simulink model "Cone_approach"  (R2024b)
settings: Solver=ode4  StartTime=0.0  StopTime=6000  FixedStep=0.01  RelTol=1e-3
values from neighbouring files (symbols this model uses):
  A = ly*lz    (= 0.25)    [Main.m]
  CD = 2.2    [Main.m]
  deltaVx_CA = 0.15    [Main.m]
  dp0_CA = dpf_RB    [Main.m]
  Dt = 0.01    [Main.m]
  Dt_con = 0.02    [Main.m]
  Dt_guid = 1    [Main.m]
  dx_max = 0.1    [Main.m]
  Ka = 1    [Main.m]
  kf = 4    [Main.m]
  landa_CA = 1.001    [Main.m]
  landa_CA_APF = 0.01    [Main.m]
  m_c0 = 50    [Main.m]
  omega_target = (mu/r_target^3)^0.5    (= 0.00113136572666)    [Main.m]
  p0_CA = pf_RB    [Main.m]
  pf_id = [-4 0 0]    [Main.m]
  rho = 1*10^(-12)    (= 1e-12)    [Main.m]
  S_CA = 0.35    [Main.m]
  S_CA_APF = 0.01    [Main.m]
  T1_CA = 10    [Main.m]
  T2_CA = T1_CA + deltax_CA/deltaVx_CA    [Main.m]
  tau = -ton/(log(1-(Uon-Uoff)/(Tmax*kf)))    [Main.m]
  Total_max_thrust = n*Tmax    (= 2)    [Main.m]
  Uoff = 0.7    [Main.m]
  Uon = 1    [Main.m]
  Vx = omega_target*r_target    (= 7668.56094333)    [Main.m]
undefined symbols (not defined in the file or in its folder): Fext
settings Model: Creator=corte  LastModifiedBy=aless

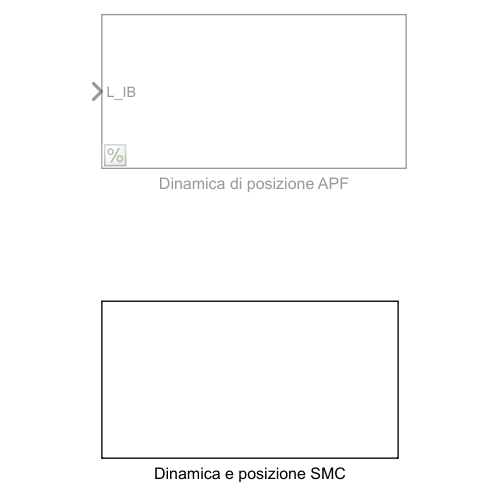
[thumbnail: Simulink's stored preview of the top-level diagram]
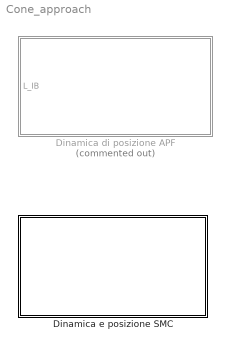
== system Cone_approach ==
  Dinamica di posizione APF : Subsystem  Commented=on
  Dinamica e posizione SMC : Subsystem

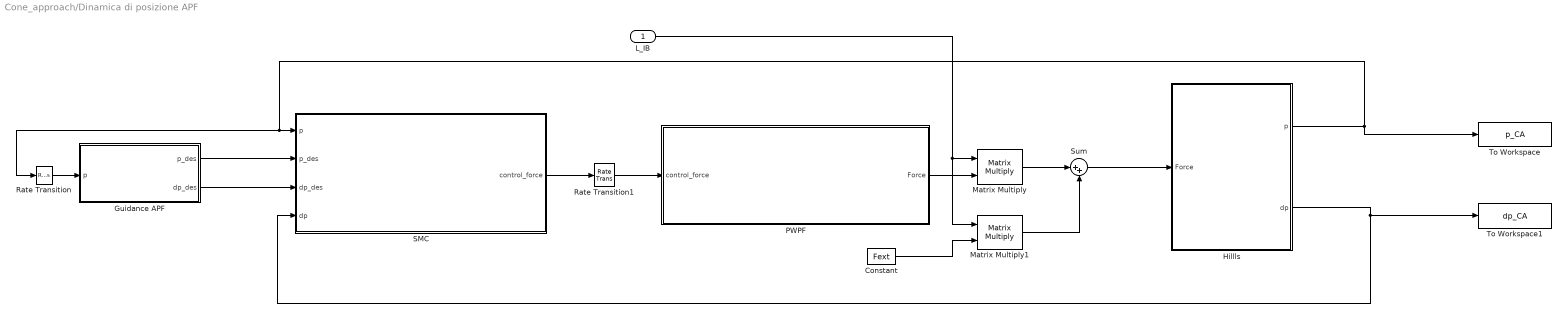
== system Cone_approach/Dinamica di posizione APF ==
  L_IB : Inport
  Constant : Constant  Value=Fext
  Guidance APF : Subsystem
  Hillls : Subsystem
  Matrix Multiply : Product  Multiplication=Matrix(*)
  Matrix Multiply1 : Product  Multiplication=Matrix(*)
  PWPF : Subsystem
  Rate Transition : RateTransition  InitialCondition=Dt  OutPortSampleTime=Dt_guid
  Rate Transition1 : RateTransition  InitialCondition=Dt_con  OutPortSampleTime=Dt
  SMC : Subsystem
  Sum : Sum  Inputs=|++
  To Workspace : ToWorkspace  VariableName=p_CA  SaveFormat=Timeseries  SampleTime=-1
  To Workspace1 : ToWorkspace  VariableName=dp_CA  SaveFormat=Timeseries  SampleTime=-1
  wires:
  Guidance APF/2(dp_des) -> SMC/3(dp_des)
  Hillls/1(p) -> To Workspace/1, Rate Transition/1, SMC/1(p)
  Guidance APF/1(p_des) -> SMC/2(p_des)
  Hillls/2(dp) -> SMC/4(dp), To Workspace1/1
  SMC/1(control_force) -> Rate Transition1/1
  Rate Transition/1 -> Guidance APF/1(p)
  Rate Transition1/1 -> PWPF/1(control_force)
  PWPF/1(Force) -> Matrix Multiply/2
  Matrix Multiply/1 -> Sum/1
  Sum/1 -> Hillls/1(Force)
  L_IB/1 -> Matrix Multiply1/1, Matrix Multiply/1
  Constant/1 -> Matrix Multiply1/2
  Matrix Multiply1/1 -> Sum/2

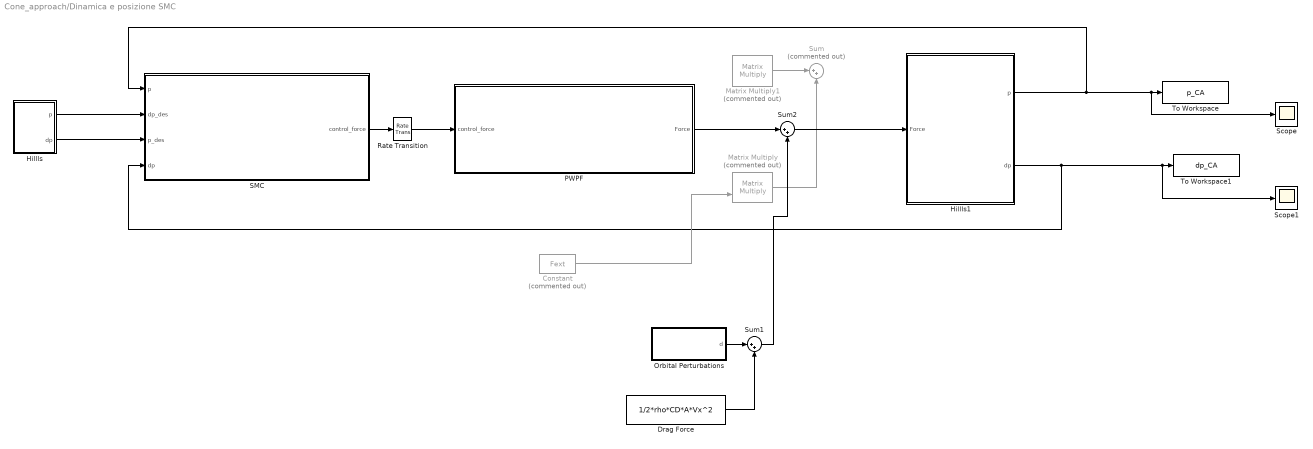
== system Cone_approach/Dinamica e posizione SMC ==
  Constant : Constant  Commented=on  Value=Fext
  Drag Force : Constant  Value=1/2*rho*CD*A*Vx^2
  Hillls : Subsystem
  Hillls1 : Subsystem
  Matrix Multiply : Product  Commented=on  Multiplication=Matrix(*)
  Matrix Multiply1 : Product  Commented=on  Multiplication=Matrix(*)
  Orbital Perturbations : Subsystem
  PWPF : Subsystem
  Rate Transition : RateTransition  InitialCondition=Dt_con  OutPortSampleTime=Dt_guid
  SMC : Subsystem
  Scope : Scope
  Scope1 : Scope
  Sum : Sum  Commented=on  Inputs=|++
  Sum1 : Sum  Inputs=|++
  Sum2 : Sum  Inputs=|++
  To Workspace : ToWorkspace  VariableName=p_CA  SaveFormat=Timeseries  SampleTime=-1
  To Workspace1 : ToWorkspace  VariableName=dp_CA  SaveFormat=Timeseries  SampleTime=-1
  wires:
  Hillls1/1(p) -> Scope/1, To Workspace/1, SMC/1(p)
  Hillls1/2(dp) -> Scope1/1, To Workspace1/1, SMC/4(dp)
  Hillls/1(p) -> SMC/2(dp_des)
  SMC/1(control_force) -> Rate Transition/1
  Hillls/2(dp) -> SMC/3(p_des)
  Rate Transition/1 -> PWPF/1(control_force)
  Constant/1 -> Matrix Multiply/2
  ? -> Matrix Multiply/1, Matrix Multiply1/1  "Aggiungere output controllo"
  Matrix Multiply/1 -> Sum/2
  Matrix Multiply1/1 -> Sum/1
  Sum1/1 -> Sum2/2
  Drag Force/1 -> Sum1/2
  Orbital Perturbations/1(d) -> Sum1/1
  PWPF/1(Force) -> Sum2/1
  Sum2/1 -> Hillls1/1(Force)

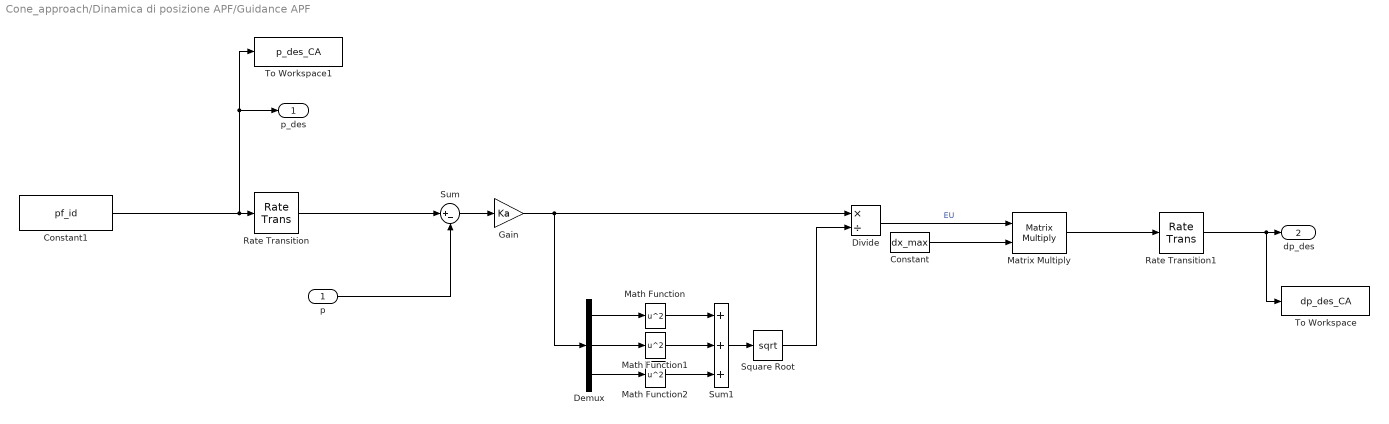
== system Cone_approach/Dinamica di posizione APF/Guidance APF ==
  p : Inport
  Constant : Constant  Value=dx_max
  Constant1 : Constant  Value=pf_id
  Demux : Demux  Outputs=3
  Divide : Product  Inputs=*/
  Gain : Gain  Gain=Ka
  Math Function : Math  Operator=square
  Math Function1 : Math  Operator=square
  Math Function2 : Math  Operator=square
  Matrix Multiply : Product  Multiplication=Matrix(*)
  Rate Transition : RateTransition  InitialCondition=Dt  OutPortSampleTime=Dt_guid
  Rate Transition1 : RateTransition  InitialCondition=Dt_guid  OutPortSampleTime=Dt
  Square Root : Sqrt
  Sum : Sum  Inputs=|+-
  Sum1 : Sum  Inputs=+++
  To Workspace : ToWorkspace  VariableName=dp_des_CA  SaveFormat=Timeseries  SampleTime=-1
  To Workspace1 : ToWorkspace  VariableName=p_des_CA  SaveFormat=Timeseries  SampleTime=-1
  p_des : Outport
  dp_des : Outport  Port=2
  wires:
  Sum/1 -> Gain/1
  p/1 -> Sum/2
  Rate Transition/1 -> Sum/1
  Constant1/1 -> To Workspace1/1, p_des/1, Rate Transition/1
  Gain/1 -> Demux/1, Divide/1
  Demux/1 -> Math Function/1
  Demux/2 -> Math Function1/1
  Demux/3 -> Math Function2/1
  Math Function/1 -> Sum1/1
  Math Function1/1 -> Sum1/2
  Math Function2/1 -> Sum1/3
  Sum1/1 -> Square Root/1
  Square Root/1 -> Divide/2
  Divide/1 -> Matrix Multiply/1  "EU"
  Constant/1 -> Matrix Multiply/2
  Matrix Multiply/1 -> Rate Transition1/1
  Rate Transition1/1 -> To Workspace/1, dp_des/1

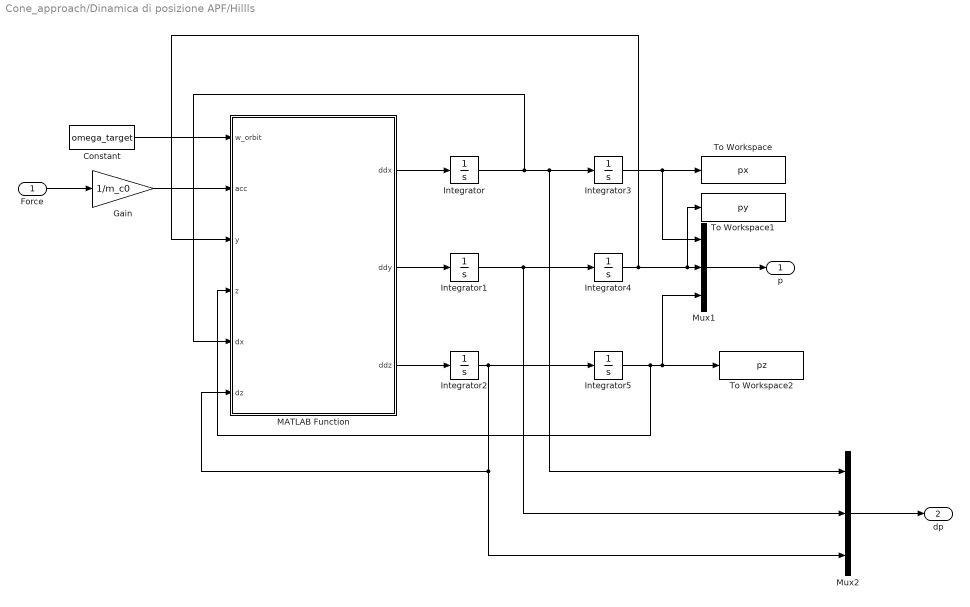
== system Cone_approach/Dinamica di posizione APF/Hillls ==
  Force : Inport
  Constant : Constant  Value=omega_target
  Gain : Gain  Gain=1/m_c0
  Integrator : Integrator  InitialCondition=dp0_CA(1)
  Integrator1 : Integrator  InitialCondition=dp0_CA(2)
  Integrator2 : Integrator  InitialCondition=dp0_CA(3)
  Integrator3 : Integrator  InitialCondition=p0_CA(1)
  Integrator4 : Integrator  InitialCondition=p0_CA(2)
  Integrator5 : Integrator  InitialCondition=p0_CA(3)
  MATLAB Function : MATLAB Function  TreatAsAtomicUnit=on
  Mux1 : Mux  Inputs=3
  Mux2 : Mux  Inputs=3
  To Workspace : ToWorkspace  VariableName=px  SaveFormat=Timeseries  SampleTime=-1
  To Workspace1 : ToWorkspace  VariableName=py  SaveFormat=Timeseries  SampleTime=-1
  To Workspace2 : ToWorkspace  VariableName=pz  SaveFormat=Timeseries  SampleTime=-1
  p : Outport
  dp : Outport  Port=2
  wires:
  Force/1 -> Gain/1
  Gain/1 -> MATLAB Function/2(acc)
  Constant/1 -> MATLAB Function/1(w_orbit)
  MATLAB Function/1(ddx) -> Integrator/1
  Integrator4/1 -> To Workspace1/1, Mux1/2, MATLAB Function/3(y)
  Integrator3/1 -> Mux1/1, To Workspace/1
  Integrator5/1 -> To Workspace2/1, Mux1/3, MATLAB Function/4(z)
  Integrator2/1 -> Integrator5/1, Mux2/3, MATLAB Function/6(dz)
  Integrator/1 -> Mux2/1, Integrator3/1, MATLAB Function/5(dx)
  MATLAB Function/2(ddy) -> Integrator1/1
  Integrator1/1 -> Mux2/2, Integrator4/1
  MATLAB Function/3(ddz) -> Integrator2/1
  Mux1/1 -> p/1
  Mux2/1 -> dp/1

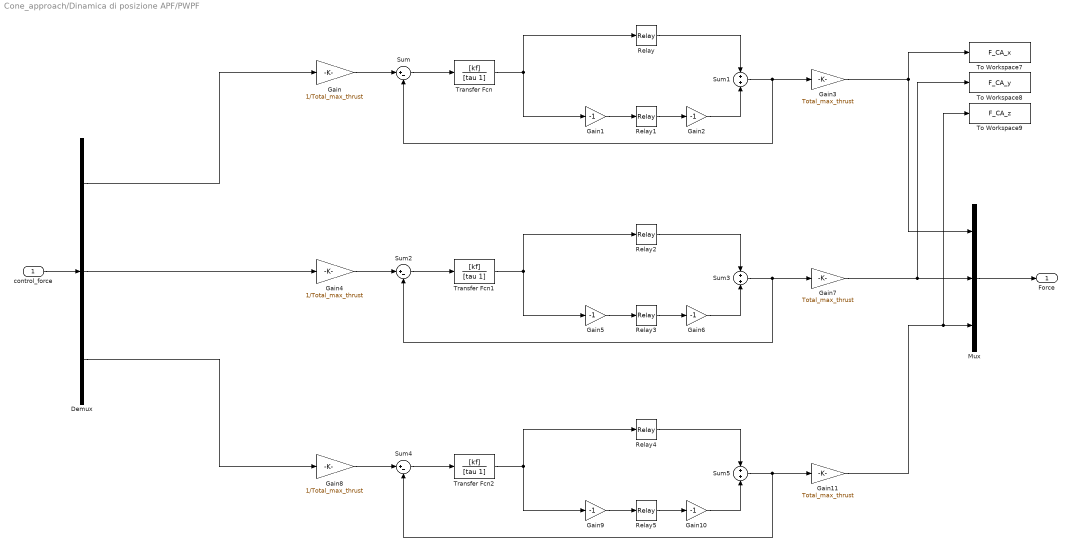
== system Cone_approach/Dinamica di posizione APF/PWPF ==
  control_force : Inport
  Demux : Demux  Outputs=3
  Gain : Gain  Gain=1/Total_max_thrust
  Gain{1..2,5..6,9..10} (6 alike) : Gain  Gain=-1
  Gain11 : Gain  Gain=Total_max_thrust
  Gain3 : Gain  Gain=Total_max_thrust
  Gain4 : Gain  Gain=1/Total_max_thrust
  Gain7 : Gain  Gain=Total_max_thrust
  Gain8 : Gain  Gain=1/Total_max_thrust
  Mux : Mux  Inputs=3
  Relay{,1..5} (6 alike) : Relay  OnSwitchValue=Uon  OffSwitchValue=Uoff
  Sum : Sum  Inputs=|+-
  Sum1 : Sum
  Sum2 : Sum  Inputs=|+-
  Sum3 : Sum
  Sum4 : Sum  Inputs=|+-
  Sum5 : Sum
  To Workspace7 : ToWorkspace  VariableName=F_CA_x  SaveFormat=Timeseries  SampleTime=-1
  To Workspace8 : ToWorkspace  VariableName=F_CA_y  SaveFormat=Timeseries  SampleTime=-1
  To Workspace9 : ToWorkspace  VariableName=F_CA_z  SaveFormat=Timeseries  SampleTime=-1
  Transfer Fcn : TransferFcn  Numerator=[kf]  Denominator=[tau 1]
  Transfer Fcn1 : TransferFcn  Numerator=[kf]  Denominator=[tau 1]
  Transfer Fcn2 : TransferFcn  Numerator=[kf]  Denominator=[tau 1]
  Force : Outport
  wires:
  Gain/1 -> Sum/1
  Gain1/1 -> Relay1/1
  Relay1/1 -> Gain2/1
  Relay/1 -> Sum1/1
  Gain2/1 -> Sum1/2
  Sum1/1 -> Sum/2, Gain3/1
  Sum/1 -> Transfer Fcn/1
  Transfer Fcn/1 -> Gain1/1, Relay/1
  control_force/1 -> Demux/1
  Demux/1 -> Gain/1
  Sum3/1 -> Sum2/2, Gain7/1
  Relay3/1 -> Gain6/1
  Gain5/1 -> Relay3/1
  Relay2/1 -> Sum3/1
  Gain4/1 -> Sum2/1
  Transfer Fcn1/1 -> Gain5/1, Relay2/1
  Demux/2 -> Gain4/1
  Sum2/1 -> Transfer Fcn1/1
  Gain6/1 -> Sum3/2
  Sum5/1 -> Sum4/2, Gain11/1
  Relay5/1 -> Gain10/1
  Gain9/1 -> Relay5/1
  Relay4/1 -> Sum5/1
  Gain8/1 -> Sum4/1
  Transfer Fcn2/1 -> Gain9/1, Relay4/1
  Demux/3 -> Gain8/1
  Sum4/1 -> Transfer Fcn2/1
  Gain10/1 -> Sum5/2
  Mux/1 -> Force/1
  Gain7/1 -> To Workspace8/1, Mux/2
  Gain3/1 -> To Workspace7/1, Mux/1
  Gain11/1 -> To Workspace9/1, Mux/3

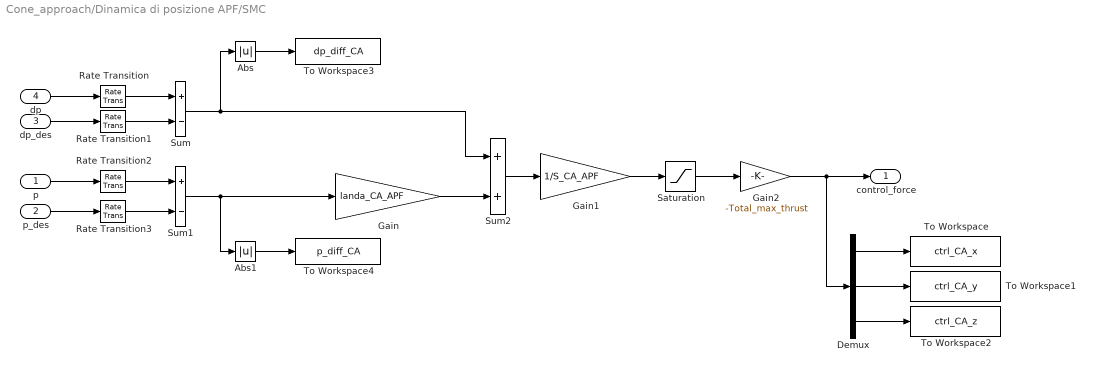
== system Cone_approach/Dinamica di posizione APF/SMC ==
  p : Inport
  p_des : Inport  Port=2
  dp_des : Inport  Port=3
  dp : Inport  Port=4
  Abs : Abs  SaturateOnIntegerOverflow=off
  Abs1 : Abs  SaturateOnIntegerOverflow=off
  Demux : Demux  Outputs=3
  Gain : Gain  Gain=landa_CA_APF
  Gain1 : Gain  Gain=1/S_CA_APF
  Gain2 : Gain  Gain=-Total_max_thrust
  Rate Transition{,1..3} (4 alike) : RateTransition  InitialCondition=Dt  OutPortSampleTime=Dt_con
  Saturation : Saturate  UpperLimit=1  LowerLimit=-1
  Sum : Sum  Inputs=+-
  Sum1 : Sum  Inputs=+-
  Sum2 : Sum
  To Workspace : ToWorkspace  VariableName=ctrl_CA_x  SaveFormat=Timeseries  SampleTime=-1
  To Workspace1 : ToWorkspace  VariableName=ctrl_CA_y  SaveFormat=Timeseries  SampleTime=-1
  To Workspace2 : ToWorkspace  VariableName=ctrl_CA_z  SaveFormat=Timeseries  SampleTime=-1
  To Workspace3 : ToWorkspace  VariableName=dp_diff_CA  SaveFormat=Timeseries  SampleTime=-1
  To Workspace4 : ToWorkspace  VariableName=p_diff_CA  SaveFormat=Timeseries  SampleTime=-1
  control_force : Outport
  wires:
  dp/1 -> Rate Transition/1
  dp_des/1 -> Rate Transition1/1
  p/1 -> Rate Transition2/1
  p_des/1 -> Rate Transition3/1
  Sum1/1 -> Abs1/1, Gain/1
  Gain/1 -> Sum2/2
  Sum/1 -> Abs/1, Sum2/1
  Sum2/1 -> Gain1/1
  Gain1/1 -> Saturation/1
  Saturation/1 -> Gain2/1
  Gain2/1 -> control_force/1, Demux/1
  Rate Transition/1 -> Sum/1
  Rate Transition1/1 -> Sum/2
  Rate Transition2/1 -> Sum1/1
  Rate Transition3/1 -> Sum1/2
  Demux/1 -> To Workspace/1
  Demux/2 -> To Workspace1/1
  Demux/3 -> To Workspace2/1
  Abs/1 -> To Workspace3/1
  Abs1/1 -> To Workspace4/1

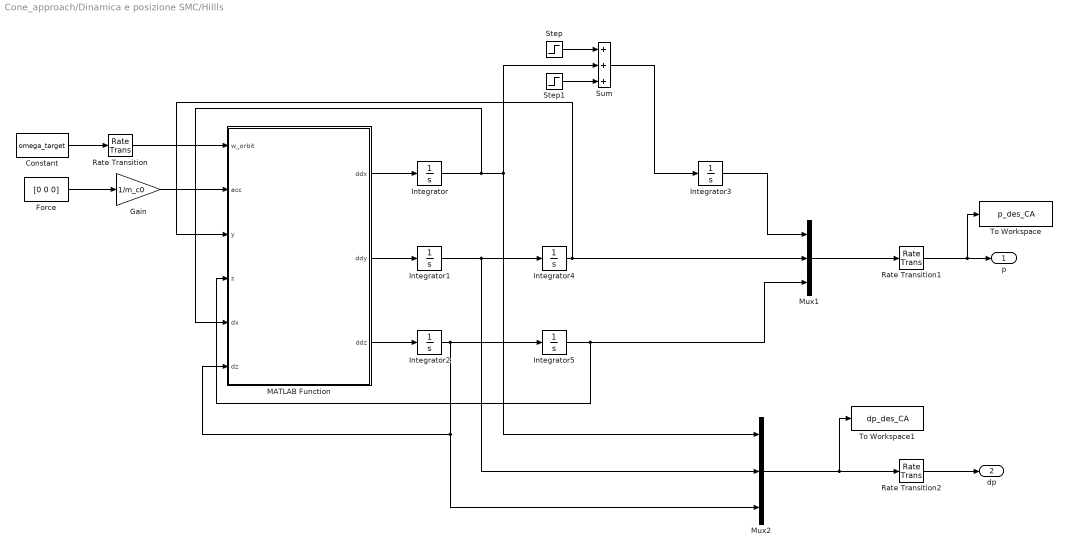
== system Cone_approach/Dinamica e posizione SMC/Hillls ==
  Constant : Constant  Value=omega_target
  Force : Constant  Value=[0 0 0]
  Gain : Gain  Gain=1/m_c0
  Integrator : Integrator  InitialCondition=dp0_CA(1)
  Integrator1 : Integrator  InitialCondition=dp0_CA(2)
  Integrator2 : Integrator  InitialCondition=dp0_CA(3)
  Integrator3 : Integrator  InitialCondition=p0_CA(1)
  Integrator4 : Integrator  InitialCondition=p0_CA(2)
  Integrator5 : Integrator  InitialCondition=p0_CA(3)
  MATLAB Function : MATLAB Function  TreatAsAtomicUnit=on
  Mux1 : Mux  Inputs=3
  Mux2 : Mux  Inputs=3
  Rate Transition : RateTransition  InitialCondition=Dt  OutPortSampleTime=Dt_guid
  Rate Transition1 : RateTransition  InitialCondition=Dt_guid  OutPortSampleTime=Dt
  Rate Transition2 : RateTransition  InitialCondition=Dt_guid  OutPortSampleTime=Dt
  Step : Step  Time=T1_CA  After=deltaVx_CA  SampleTime=0
  Step1 : Step  Time=T2_CA  After=-deltaVx_CA  SampleTime=0
  Sum : Sum  Inputs=+++
  To Workspace : ToWorkspace  VariableName=p_des_CA  SaveFormat=Timeseries  SampleTime=-1
  To Workspace1 : ToWorkspace  VariableName=dp_des_CA  SaveFormat=Timeseries  SampleTime=-1
  p : Outport
  dp : Outport  Port=2
  wires:
  Force/1 -> Gain/1
  Gain/1 -> MATLAB Function/2(acc)
  Constant/1 -> Rate Transition/1
  MATLAB Function/1(ddx) -> Integrator/1
  Integrator4/1 -> Mux1/2, MATLAB Function/3(y)
  Integrator3/1 -> Mux1/1
  Integrator5/1 -> Mux1/3, MATLAB Function/4(z)
  Integrator2/1 -> Integrator5/1, Mux2/3, MATLAB Function/6(dz)
  Integrator/1 -> Mux2/1, Sum/2, MATLAB Function/5(dx)
  MATLAB Function/2(ddy) -> Integrator1/1
  Integrator1/1 -> Mux2/2, Integrator4/1
  MATLAB Function/3(ddz) -> Integrator2/1
  Mux1/1 -> Rate Transition1/1
  Mux2/1 -> To Workspace1/1, Rate Transition2/1
  Step/1 -> Sum/1
  Step1/1 -> Sum/3
  Sum/1 -> Integrator3/1
  Rate Transition/1 -> MATLAB Function/1(w_orbit)
  Rate Transition1/1 -> To Workspace/1, p/1
  Rate Transition2/1 -> dp/1

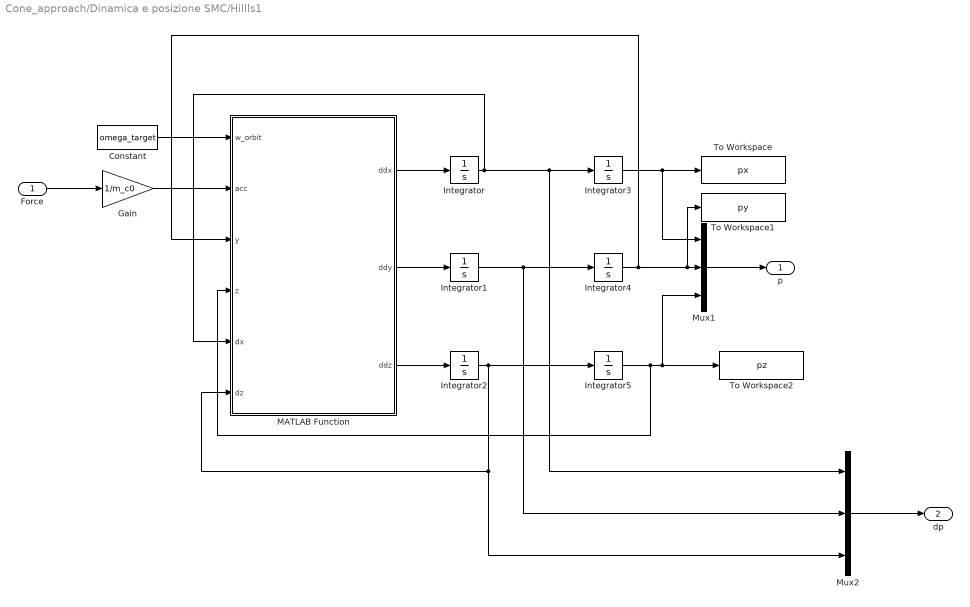
== system Cone_approach/Dinamica e posizione SMC/Hillls1 ==
  Force : Inport
  Constant : Constant  Value=omega_target
  Gain : Gain  Gain=1/m_c0
  Integrator : Integrator  InitialCondition=dp0_CA(1)
  Integrator1 : Integrator  InitialCondition=dp0_CA(2)
  Integrator2 : Integrator  InitialCondition=dp0_CA(3)
  Integrator3 : Integrator  InitialCondition=p0_CA(1)
  Integrator4 : Integrator  InitialCondition=p0_CA(2)
  Integrator5 : Integrator  InitialCondition=p0_CA(3)
  MATLAB Function : MATLAB Function  TreatAsAtomicUnit=on
  Mux1 : Mux  Inputs=3
  Mux2 : Mux  Inputs=3
  To Workspace : ToWorkspace  VariableName=px  SaveFormat=Timeseries  SampleTime=-1
  To Workspace1 : ToWorkspace  VariableName=py  SaveFormat=Timeseries  SampleTime=-1
  To Workspace2 : ToWorkspace  VariableName=pz  SaveFormat=Timeseries  SampleTime=-1
  p : Outport
  dp : Outport  Port=2
  wires:
  Force/1 -> Gain/1
  Gain/1 -> MATLAB Function/2(acc)
  MATLAB Function/1(ddx) -> Integrator/1
  Integrator4/1 -> To Workspace1/1, Mux1/2, MATLAB Function/3(y)
  Integrator3/1 -> Mux1/1, To Workspace/1
  Integrator5/1 -> To Workspace2/1, Mux1/3, MATLAB Function/4(z)
  Integrator2/1 -> Integrator5/1, Mux2/3, MATLAB Function/6(dz)
  Integrator/1 -> Mux2/1, Integrator3/1, MATLAB Function/5(dx)
  MATLAB Function/2(ddy) -> Integrator1/1
  Integrator1/1 -> Mux2/2, Integrator4/1
  MATLAB Function/3(ddz) -> Integrator2/1
  Mux1/1 -> p/1
  Mux2/1 -> dp/1
  Constant/1 -> MATLAB Function/1(w_orbit)

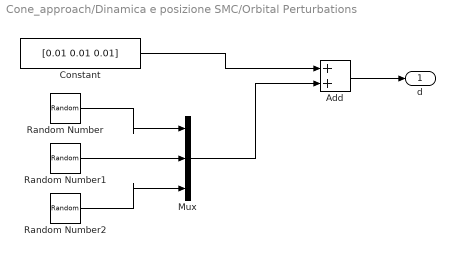
== system Cone_approach/Dinamica e posizione SMC/Orbital Perturbations ==
  Add : Sum
  Constant : Constant  Value=[0.01 0.01 0.01]
  Mux : Mux  Inputs=3
  Random Number : RandomNumber  Variance=(0.00001)^2  Seed=1  SampleTime=1
  Random Number1 : RandomNumber  Variance=(0.00001)^2  Seed=765  SampleTime=1
  Random Number2 : RandomNumber  Variance=(0.00001)^2  Seed=6  SampleTime=1
  d : Outport
  wires:
  Add/1 -> d/1
  Constant/1 -> Add/1
  Mux/1 -> Add/2
  Random Number2/1 -> Mux/3
  Random Number1/1 -> Mux/2
  Random Number/1 -> Mux/1

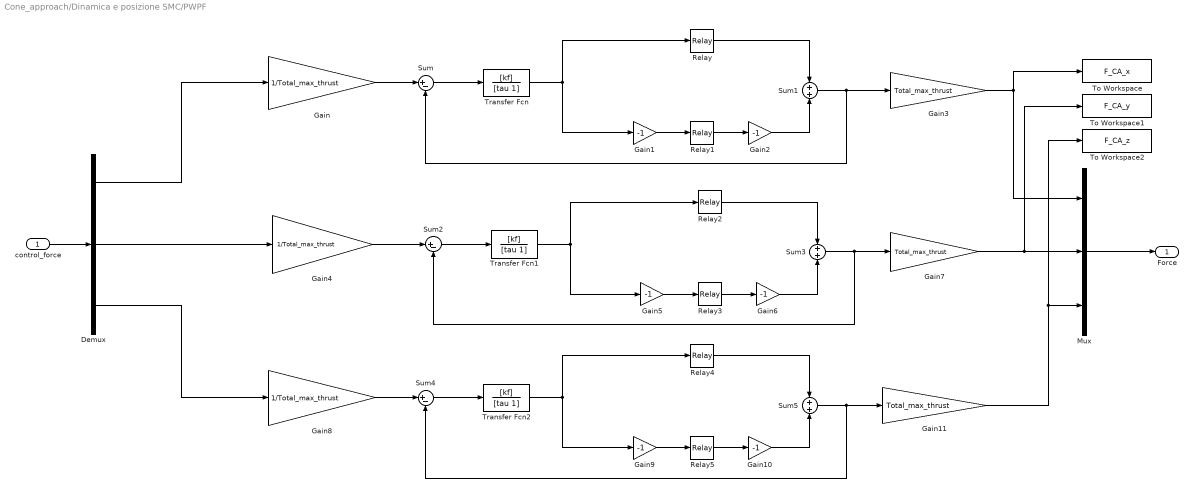
== system Cone_approach/Dinamica e posizione SMC/PWPF ==
  control_force : Inport
  Demux : Demux  Outputs=3
  Gain : Gain  Gain=1/Total_max_thrust
  Gain{1..2,5..6,9..10} (6 alike) : Gain  Gain=-1
  Gain11 : Gain  Gain=Total_max_thrust
  Gain3 : Gain  Gain=Total_max_thrust
  Gain4 : Gain  Gain=1/Total_max_thrust
  Gain7 : Gain  Gain=Total_max_thrust
  Gain8 : Gain  Gain=1/Total_max_thrust
  Mux : Mux  Inputs=3
  Relay{,1..5} (6 alike) : Relay  OnSwitchValue=Uon  OffSwitchValue=Uoff
  Sum : Sum  Inputs=|+-
  Sum1 : Sum
  Sum2 : Sum  Inputs=|+-
  Sum3 : Sum
  Sum4 : Sum  Inputs=|+-
  Sum5 : Sum
  To Workspace : ToWorkspace  VariableName=F_CA_x  SaveFormat=Timeseries  SampleTime=-1
  To Workspace1 : ToWorkspace  VariableName=F_CA_y  SaveFormat=Timeseries  SampleTime=-1
  To Workspace2 : ToWorkspace  VariableName=F_CA_z  SaveFormat=Timeseries  SampleTime=-1
  Transfer Fcn : TransferFcn  Numerator=[kf]  Denominator=[tau 1]
  Transfer Fcn1 : TransferFcn  Numerator=[kf]  Denominator=[tau 1]
  Transfer Fcn2 : TransferFcn  Numerator=[kf]  Denominator=[tau 1]
  Force : Outport
  wires:
  Gain/1 -> Sum/1
  Gain1/1 -> Relay1/1
  Relay1/1 -> Gain2/1
  Relay/1 -> Sum1/1
  Gain2/1 -> Sum1/2
  Sum1/1 -> Sum/2, Gain3/1
  Gain3/1 -> To Workspace/1, Mux/1
  Sum/1 -> Transfer Fcn/1
  Transfer Fcn/1 -> Gain1/1, Relay/1
  control_force/1 -> Demux/1
  Demux/1 -> Gain/1
  Sum3/1 -> Sum2/2, Gain7/1
  Relay3/1 -> Gain6/1
  Gain7/1 -> To Workspace1/1, Mux/2
  Gain5/1 -> Relay3/1
  Relay2/1 -> Sum3/1
  Gain4/1 -> Sum2/1
  Transfer Fcn1/1 -> Gain5/1, Relay2/1
  Demux/2 -> Gain4/1
  Sum2/1 -> Transfer Fcn1/1
  Gain6/1 -> Sum3/2
  Sum5/1 -> Sum4/2, Gain11/1
  Relay5/1 -> Gain10/1
  Gain11/1 -> To Workspace2/1, Mux/3
  Gain9/1 -> Relay5/1
  Relay4/1 -> Sum5/1
  Gain8/1 -> Sum4/1
  Transfer Fcn2/1 -> Gain9/1, Relay4/1
  Demux/3 -> Gain8/1
  Sum4/1 -> Transfer Fcn2/1
  Gain10/1 -> Sum5/2
  Mux/1 -> Force/1

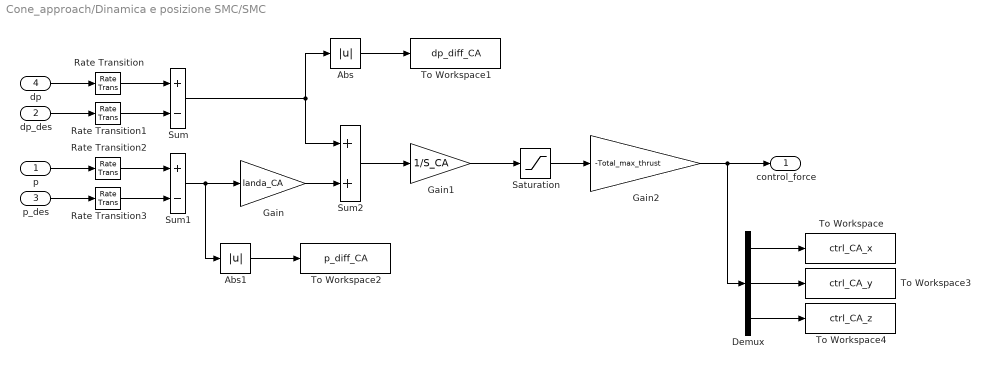
== system Cone_approach/Dinamica e posizione SMC/SMC ==
  p : Inport
  dp_des : Inport  Port=2
  p_des : Inport  Port=3
  dp : Inport  Port=4
  Abs : Abs  SaturateOnIntegerOverflow=off
  Abs1 : Abs  SaturateOnIntegerOverflow=off
  Demux : Demux  Outputs=3
  Gain : Gain  Gain=landa_CA
  Gain1 : Gain  Gain=1/S_CA
  Gain2 : Gain  Gain=-Total_max_thrust
  Rate Transition{,1..3} (4 alike) : RateTransition  InitialCondition=Dt  OutPortSampleTime=Dt_con
  Saturation : Saturate  UpperLimit=1  LowerLimit=-1
  Sum : Sum  Inputs=+-
  Sum1 : Sum  Inputs=+-
  Sum2 : Sum
  To Workspace : ToWorkspace  VariableName=ctrl_CA_x  SaveFormat=Timeseries  SampleTime=-1
  To Workspace1 : ToWorkspace  VariableName=dp_diff_CA  SaveFormat=Timeseries  SampleTime=-1
  To Workspace2 : ToWorkspace  VariableName=p_diff_CA  SaveFormat=Timeseries  SampleTime=-1
  To Workspace3 : ToWorkspace  VariableName=ctrl_CA_y  SaveFormat=Timeseries  SampleTime=-1
  To Workspace4 : ToWorkspace  VariableName=ctrl_CA_z  SaveFormat=Timeseries  SampleTime=-1
  control_force : Outport
  wires:
  dp/1 -> Rate Transition/1
  dp_des/1 -> Rate Transition1/1
  p/1 -> Rate Transition2/1
  p_des/1 -> Rate Transition3/1
  Sum1/1 -> Abs1/1, Gain/1
  Gain/1 -> Sum2/2
  Sum/1 -> Abs/1, Sum2/1
  Sum2/1 -> Gain1/1
  Gain1/1 -> Saturation/1
  Saturation/1 -> Gain2/1
  Abs/1 -> To Workspace1/1
  Abs1/1 -> To Workspace2/1
  Rate Transition/1 -> Sum/1
  Rate Transition1/1 -> Sum/2
  Rate Transition2/1 -> Sum1/1
  Rate Transition3/1 -> Sum1/2
  Demux/1 -> To Workspace/1
  Gain2/1 -> Demux/1, control_force/1
  Demux/2 -> To Workspace3/1
  Demux/3 -> To Workspace4/1

== matlab function Cone_approach/Dinamica di posizione APF/Hillls/MATLAB Function ==
  data: w_orbit input; ddx output size=1; acc input; y input; z input; dx input; dz input; ddy output size=1; ddz output size=1
function [ddx, ddy, ddz] = fcn(w_orbit, acc, y, z, dx, dz)
ddx=acc(1)+2*w_orbit*dz;
ddy=acc(2)+w_orbit^2*y;
ddz=acc(3)+3*w_orbit^2*z-2*w_orbit*dx;

end

== matlab function Cone_approach/Dinamica e posizione SMC/Hillls/MATLAB Function ==
  data: w_orbit input; ddx output size=1; acc input; y input; z input; dx input; dz input; ddy output size=1; ddz output size=1
function [ddx, ddy, ddz] = fcn(w_orbit, acc, y, z, dx, dz)
ddx=acc(1)+2*w_orbit*dz;
ddy=acc(2)+w_orbit^2*y;
ddz=acc(3)+3*w_orbit^2*z-2*w_orbit*dx;

end

== matlab function Cone_approach/Dinamica e posizione SMC/Hillls1/MATLAB Function ==
  data: w_orbit input; ddx output size=1; acc input; y input; z input; dx input; dz input; ddy output size=1; ddz output size=1
function [ddx, ddy, ddz] = fcn(w_orbit, acc, y, z, dx, dz)
ddx=acc(1)+2*w_orbit*dz;
ddy=acc(2)+w_orbit^2*y;
ddz=acc(3)+3*w_orbit^2*z-2*w_orbit*dx;

end
